simulink model "Q7"  (Simulink 8.5)
settings: Solver=ode45  StartTime=0.0  StopTime=T  RelTol=1e-3
values from neighbouring files (symbols this model uses):
  b = 0    [e_11.m]    (also in e_12.m = 0.025; e_13.m; lab2.m)
  dy0 = dy    [e_11.m]    (also in lab2.m)
  y0 = y    [e_11.m]    (also in lab2.m)
settings Model: Creator=ricar  LastModifiedBy=Carlos
settings DataIOCC: LimitDataPoints=off  SignalLoggingSaveFormat=Dataset
settings OptimizationCC: ExpressionDepthLimit=128
settings DebuggingCC: UnderspecifiedInitializationDetection=Simplified  MergeDetectMultiDrivingBlocksExec=error  FcnCallInpInsideContextMsg=EnableAllAsError  StateNameClashWarn=none
settings HardwareCC: ProdBitPerPointer=64  ProdLargestAtomicFloat=Float  ProdIntDivRoundTo=Zero  ProdEndianess=LittleEndian  ProdHWDeviceType=Specified
settings GRTTargetCC: CombineOutputUpdateFcns=on  GRTInterface=off

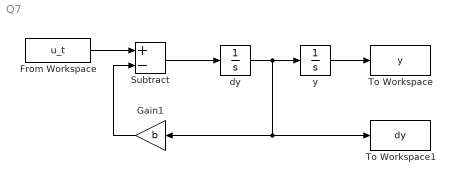
== system Q7 ==
  From Workspace : FromWorkspace  VariableName=u_t  SampleTime=0
  Gain1 : Gain  Gain=b
  Subtract : Sum  Inputs=+-
  To Workspace : ToWorkspace  VariableName=y  SampleTime=-1
  To Workspace1 : ToWorkspace  VariableName=dy  SampleTime=-1
  dy : Integrator  InitialCondition=dy0
  y : Integrator  InitialCondition=y0
  wires:
  From Workspace/1 -> Subtract/1
  Subtract/1 -> dy/1
  dy/1 -> To Workspace1/1, Gain1/1, y/1
  Gain1/1 -> Subtract/2
  y/1 -> To Workspace/1
